simulink model "Kinct_object_tracking"  (Simulink 8.5)
settings: Solver=FixedStepDiscrete  StartTime=0.0  StopTime=inf  RelTol=1e-3
undefined symbols (not defined in the file): HDTV, Rec, strel
libraries: visionsources x3, nid_lib x3, visionsinks x2, simulink x2, visiontextngfix x2, visionstatistics x1, visionconversions x1, visionmorphops x1
settings Model: Creator=Arathos  LastModifiedBy=Arathos_II
settings SolverCC: PositivePriorityOrder=on
settings DataIOCC: SignalLoggingSaveFormat=Dataset
settings OptimizationCC: EnhancedBackFolding=on  SimCompilerOptimization=on
settings DebuggingCC: AlgebraicLoopMsg=none  SolverPrmCheckMsg=warning  FcnCallInpInsideContextMsg=EnableAllAsError
settings RTWCC: RTWCompilerOptimization=on
settings GRTTargetCC: CombineOutputUpdateFcns=on  GRTInterface=off
settings ConfigComp: Description=Design Verifier Custom Configuration Component  DVMaxTestCaseSteps=500  DVTestSuiteOptimization=CombinedObjectives (Nonlinear Extended)  DVDetectActiveLogic=on

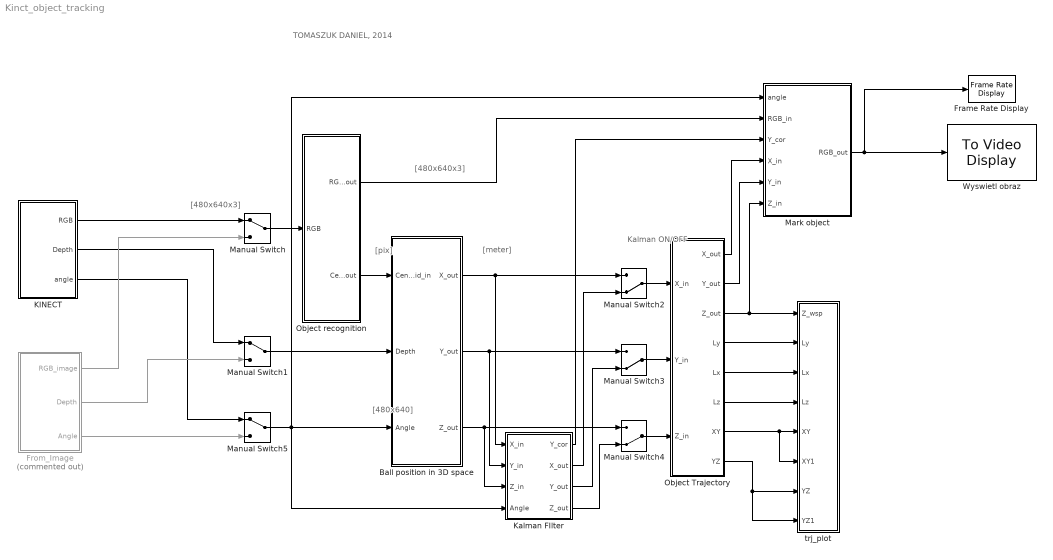
== system Kinct_object_tracking ==
  note: TOMASZUK DANIEL, 2014
  note: Kalman ON/OFF
  note: [meter]
  note: [pix]
  note: [480x640]
  note: [480x640x3]
  note: [480x640x3]
  Ball position in 3D space : Subsystem
  Frame Rate Display : visionsinks/Frame Rate Display  UpdateRate=10
  From_Image : Subsystem  Commented=on
  KINECT : Subsystem
  Kalman FIlter : Subsystem
  Manual Switch : ManualSwitch
  Manual Switch1 : ManualSwitch
  Manual Switch2 : ManualSwitch  CurrentSetting=0
  Manual Switch3 : ManualSwitch  CurrentSetting=0
  Manual Switch4 : ManualSwitch  CurrentSetting=0
  Manual Switch5 : ManualSwitch
  Mark object : Subsystem
  Object Trajectory : Subsystem
  Object recognition : Subsystem
  Wyswietl obraz : visionsinks/To Video Display  windowSizeMode=True size (1:1)  openAtMdlStart=on  fullScreen=off  videoWindowX=411  videoWindowY=172  saveWindowSize=off  videoWindowWidth=640  videoWindowHeight=480  inputColorFormat=RGB  inputType=Obsolete  imagePorts=One multidimensional signal  OutputDevice=On-screen video monitor  dataOrg=Column-major  isWindowOpen=on
  trj_plot : Subsystem
  wires:
  Object Trajectory/3(Z_out) -> trj_plot/1(Z_wsp), Mark object/6(Z_in)
  Object Trajectory/1(X_out) -> Mark object/4(X_in)
  Object Trajectory/2(Y_out) -> Mark object/5(Y_in)
  Object recognition/2(Centroid_out) -> Ball position in 3D space/1(Centroid_in)
  Object recognition/1(RGB_out) -> Mark object/2(RGB_in)
  Manual Switch5/1 -> Ball position in 3D space/3(Angle), Kalman FIlter/4(Angle), Mark object/1(angle)
  From_Image/3(Angle) -> Manual Switch5/2
  KINECT/3(angle) -> Manual Switch5/1
  From_Image/2(Depth) -> Manual Switch1/2
  KINECT/2(Depth) -> Manual Switch1/1
  From_Image/1(RGB_image) -> Manual Switch/2
  KINECT/1(RGB) -> Manual Switch/1
  Mark object/1(RGB_out) -> Wyswietl obraz/1, Frame Rate Display/1
  Manual Switch1/1 -> Ball position in 3D space/2(Depth)
  Manual Switch/1 -> Object recognition/1(RGB)
  Ball position in 3D space/1(X_out) -> Manual Switch2/1, Kalman FIlter/1(X_in)
  Ball position in 3D space/2(Y_out) -> Manual Switch3/1, Kalman FIlter/2(Y_in)
  Ball position in 3D space/3(Z_out) -> Manual Switch4/1, Kalman FIlter/3(Z_in)
  Kalman FIlter/2(X_out) -> Manual Switch2/2
  Kalman FIlter/3(Y_out) -> Manual Switch3/2
  Kalman FIlter/4(Z_out) -> Manual Switch4/2
  Kalman FIlter/1(Y_cor) -> Mark object/3(Y_cor)
  Manual Switch2/1 -> Object Trajectory/1(X_in)
  Manual Switch3/1 -> Object Trajectory/2(Y_in)
  Manual Switch4/1 -> Object Trajectory/3(Z_in)
  Object Trajectory/4(Ly) -> trj_plot/2(Ly)
  Object Trajectory/5(Lx) -> trj_plot/3(Lx)
  Object Trajectory/6(Lz) -> trj_plot/4(Lz)
  Object Trajectory/7(XY) -> trj_plot/6(XY1), trj_plot/5(XY)
  Object Trajectory/8(YZ) -> trj_plot/7(YZ), trj_plot/8(YZ1)

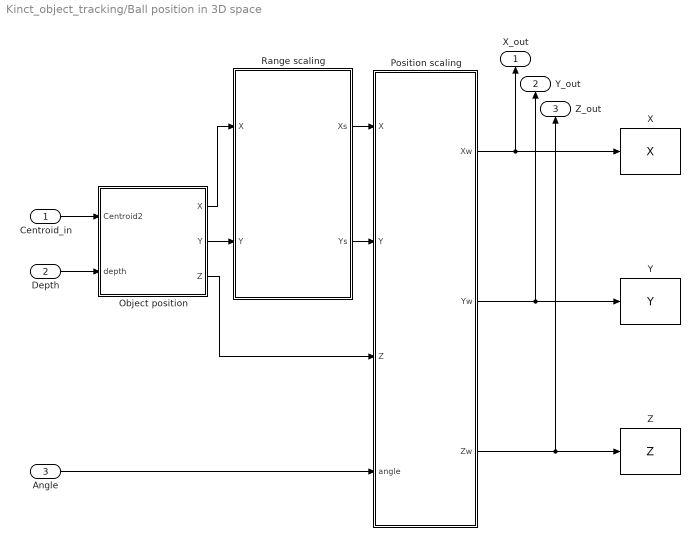
== system Kinct_object_tracking/Ball position in 3D space ==
  Centroid_in : Inport
  Depth : Inport  Port=2
  Angle : Inport  Port=3
  Object position : MATLAB Function  TreatAsAtomicUnit=on
  Position scaling : MATLAB Function  TreatAsAtomicUnit=on
  Range scaling : MATLAB Function  TreatAsAtomicUnit=on
  X : ToWorkspace  VariableName=X  SampleTime=-1
  Y : ToWorkspace  VariableName=Y  SampleTime=-1
  Z : ToWorkspace  VariableName=Z  SampleTime=-1
  X_out : Outport
  Y_out : Outport  Port=2
  Z_out : Outport  Port=3
  wires:
  Object position/3(Z) -> Position scaling/3(Z)
  Object position/1(X) -> Range scaling/1(X)
  Object position/2(Y) -> Range scaling/2(Y)
  Depth/1 -> Object position/2(depth)
  Centroid_in/1 -> Object position/1(Centroid2)
  Position scaling/3(Zw) -> Z_out/1, Z/1
  Range scaling/1(Xs) -> Position scaling/1(X)
  Position scaling/1(Xw) -> X_out/1, X/1
  Range scaling/2(Ys) -> Position scaling/2(Y)
  Position scaling/2(Yw) -> Y_out/1, Y/1
  Angle/1 -> Position scaling/4(angle)

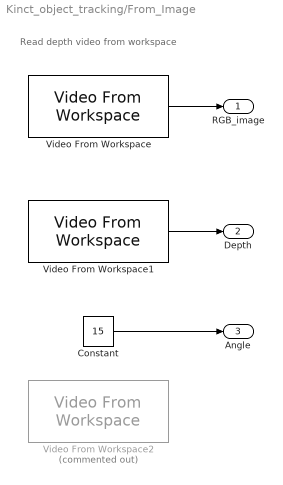
== system Kinct_object_tracking/From_Image ==
  note: Read depth video from workspace
  Constant : Constant  Value=15
  Video From Workspace : visionsources/Video From Workspace  signal=RGB  Ts=0.03333333333333333  finalout=Obsolete  finaloutActive=Holding final value  imagePorts=One multidimensional signal  OutPortLabels=R|G|B
  Video From Workspace1 : visionsources/Video From Workspace  signal=Depth  Ts=0.03333333333333333  finalout=Obsolete  finaloutActive=Holding final value  imagePorts=One multidimensional signal  OutPortLabels=R|G|B
  Video From Workspace2 : visionsources/Video From Workspace  Commented=on  signal=Depth_image  Ts=0.03333333333333333  finalout=Obsolete  finaloutActive=Holding final value  imagePorts=One multidimensional signal  OutPortLabels=R|G|B
  RGB_image : Outport
  Depth : Outport  Port=2
  Angle : Outport  Port=3
  wires:
  Video From Workspace/1 -> RGB_image/1
  Video From Workspace1/1 -> Depth/1
  Constant/1 -> Angle/1

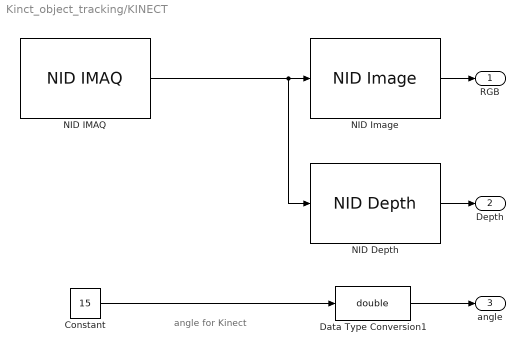
== system Kinct_object_tracking/KINECT ==
  note: angle for Kinect
  Constant : Constant  Value=15
  Data Type Conversion1 : DataTypeConversion  OutDataTypeStr=double  RndMeth=Round
  NID Depth : nid_lib/NID Depth  depthOutput=Depth  conv_XYZ_RW=on  viewer=off
  NID IMAQ : nid_lib/NID IMAQ  imaq_depth=on  imaq_motion=off  imaq_image=on  view_point=on  imaq_skeleton=off  imaq_ir=off  mirror_image=off  imaq_sample_time=1/30  res_fps=QVGA (320x240): 60 FPS  needPsiPose=off  angle_input=off  angle=15  angle_read=off  near_mode=off  seated_mode=off  skeleton_smooth=[0.5 0.5 0.5 0.05 0.04]  infer_skeleton=off
  NID Image : nid_lib/NID Image  imageOutput=RGB
  RGB : Outport
  Depth : Outport  Port=2
  angle : Outport  Port=3
  wires:
  NID IMAQ/1 -> NID Depth/1, NID Image/1
  NID Image/1 -> RGB/1
  Data Type Conversion1/1 -> angle/1
  Constant/1 -> Data Type Conversion1/1
  NID Depth/1 -> Depth/1

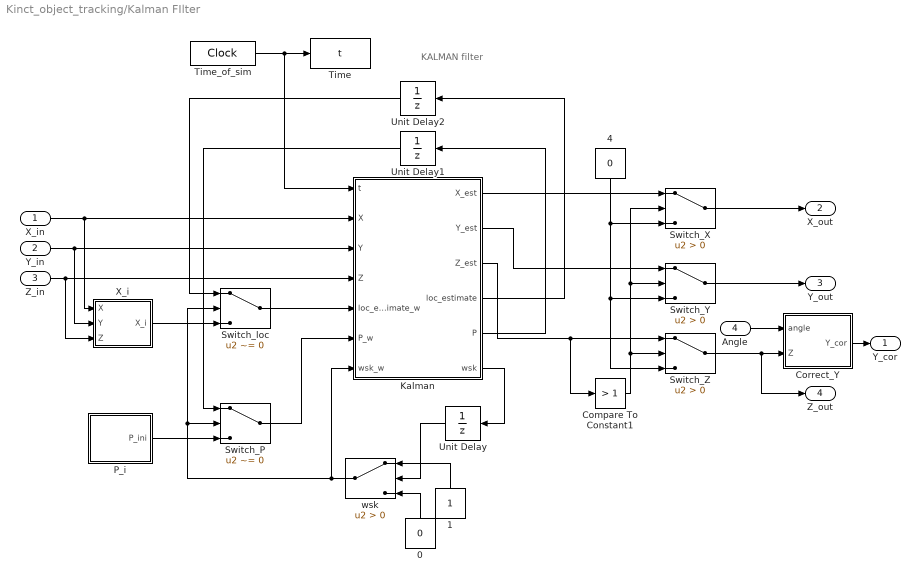
== system Kinct_object_tracking/Kalman FIlter ==
  note: KALMAN filter
  X_in : Inport
  Y_in : Inport  Port=2
  Z_in : Inport  Port=3
  Angle : Inport  Port=4
  0 : Constant  Value=0
  1 : Constant
  4 : Constant  Value=0
  Compare To Constant1 : simulink/Logic and Bit Operations/Compare To Constant  relop=>  const=1  OutDataTypeStr=boolean
  Correct_Y : MATLAB Function  TreatAsAtomicUnit=on
  Kalman : MATLAB Function  TreatAsAtomicUnit=on
  P_i : MATLAB Function  TreatAsAtomicUnit=on
  Switch_P : Switch  Criteria=u2 ~= 0
  Switch_X : Switch  Criteria=u2 > Threshold
  Switch_Y : Switch  Criteria=u2 > Threshold
  Switch_Z : Switch  Criteria=u2 > Threshold
  Switch_loc : Switch  Criteria=u2 ~= 0
  Time : ToWorkspace  VariableName=t  SampleTime=-1
  Time_of_sim : DigitalClock  SampleTime=0.0333333333333333333333333
  Unit Delay : UnitDelay  SampleTime=-1
  Unit Delay1 : UnitDelay  SampleTime=-1
  Unit Delay2 : UnitDelay  SampleTime=-1
  X_i : MATLAB Function  TreatAsAtomicUnit=on
  wsk : Switch  Criteria=u2 > Threshold
  Y_cor : Outport
  X_out : Outport  Port=2
  Y_out : Outport  Port=3
  Z_out : Outport  Port=4
  wires:
  Z_in/1 -> Kalman/4(Z), X_i/3(Z)
  X_in/1 -> X_i/1(X), Kalman/2(X)
  Time_of_sim/1 -> Kalman/1(t), Time/1
  Kalman/4(loc_estimate) -> Unit Delay2/1
  Kalman/5(P) -> Unit Delay1/1
  Kalman/6(wsk) -> Unit Delay/1
  Unit Delay/1 -> wsk/2
  wsk/1 -> Switch_P/2, Switch_loc/2, Kalman/7(wsk_w)
  0/1 -> wsk/3
  1/1 -> wsk/1
  Switch_P/1 -> Kalman/6(P_w)
  P_i/1(P_ini) -> Switch_P/3
  Unit Delay1/1 -> Switch_P/1
  X_i/1(X_i) -> Switch_loc/3
  Switch_loc/1 -> Kalman/5(loc_estimate_w)
  Unit Delay2/1 -> Switch_loc/1
  Y_in/1 -> X_i/2(Y), Kalman/3(Y)
  Switch_X/1 -> X_out/1
  Switch_Y/1 -> Y_out/1
  Correct_Y/1(Y_cor) -> Y_cor/1
  Compare To Constant1/1 -> Switch_X/2, Switch_Y/2, Switch_Z/2
  4/1 -> Switch_Y/3, Switch_Z/3, Switch_X/3
  Angle/1 -> Correct_Y/1(angle)
  Switch_Z/1 -> Z_out/1, Correct_Y/2(Z)
  Kalman/1(X_est) -> Switch_X/1
  Kalman/2(Y_est) -> Switch_Y/1
  Kalman/3(Z_est) -> Compare To Constant1/1, Switch_Z/1

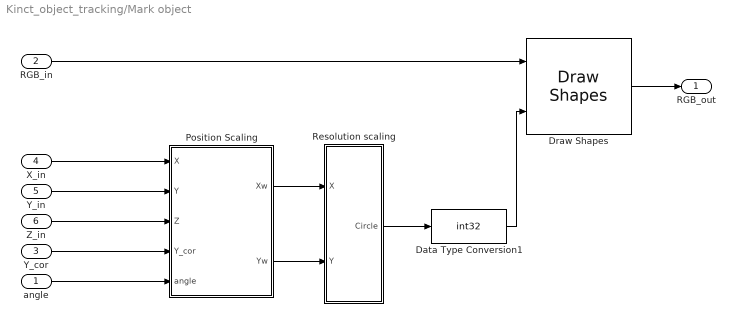
== system Kinct_object_tracking/Mark object ==
  angle : Inport
  RGB_in : Inport  Port=2
  Y_cor : Inport  Port=3
  X_in : Inport  Port=4
  Y_in : Inport  Port=5
  Z_in : Inport  Port=6
  Data Type Conversion1 : DataTypeConversion  OutDataTypeStr=int32  RndMeth=Round
  Draw Shapes : visiontextngfix/Draw Shapes  shape=Circles  fill=off  lineWidth=1  fillClrSource=Specify via dialog  display=User-specified value  intensity=200  color=[0 255 0]  opacity=0.6  viewport=Entire image  antialiasing=off  inType=Obsolete  imagePorts=One multidimensional signal  prodOutputMode=Binary point scaling  prodOutputWordLength=32  prodOutputFracLength=14  memoryMode=Specify word length  memoryWordLength=16  memoryFracLength=14  roundingMode=Floor  overflowMode=off
  Position Scaling : MATLAB Function  TreatAsAtomicUnit=on
  Resolution scaling : MATLAB Function  TreatAsAtomicUnit=on
  RGB_out : Outport
  wires:
  Y_in/1 -> Position Scaling/2(Y)
  X_in/1 -> Position Scaling/1(X)
  RGB_in/1 -> Draw Shapes/1
  Position Scaling/1(Xw) -> Resolution scaling/1(X)
  Position Scaling/2(Yw) -> Resolution scaling/2(Y)
  Resolution scaling/1(Circle) -> Data Type Conversion1/1
  Data Type Conversion1/1 -> Draw Shapes/2
  Draw Shapes/1 -> RGB_out/1
  Z_in/1 -> Position Scaling/3(Z)
  Y_cor/1 -> Position Scaling/4(Y_cor)
  angle/1 -> Position Scaling/5(angle)

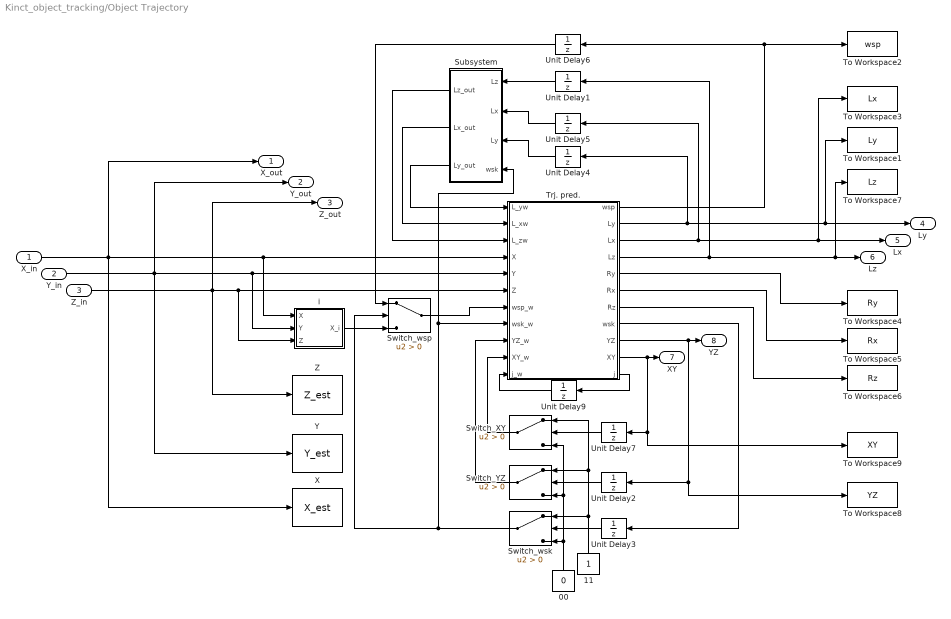
== system Kinct_object_tracking/Object Trajectory ==
  X_in : Inport
  Y_in : Inport  Port=2
  Z_in : Inport  Port=3
  00 : Constant  Value=0
  11 : Constant
  Subsystem : Subsystem
  Switch_XY : Switch  Criteria=u2 > Threshold
  Switch_YZ : Switch  Criteria=u2 > Threshold
  Switch_wsk : Switch  Criteria=u2 > Threshold
  Switch_wsp : Switch  Criteria=u2 > Threshold
  To Workspace1 : ToWorkspace  VariableName=Ly  SampleTime=-1
  To Workspace2 : ToWorkspace  VariableName=wsp  SampleTime=-1
  To Workspace3 : ToWorkspace  VariableName=Lx  SampleTime=-1
  To Workspace4 : ToWorkspace  VariableName=Ry  SampleTime=-1
  To Workspace5 : ToWorkspace  VariableName=Rx  SampleTime=-1
  To Workspace6 : ToWorkspace  VariableName=Rz  SampleTime=-1
  To Workspace7 : ToWorkspace  VariableName=Lz  SampleTime=-1
  To Workspace8 : ToWorkspace  VariableName=YZ  SampleTime=-1
  To Workspace9 : ToWorkspace  VariableName=XY  SampleTime=-1
  Trj. pred. : MATLAB Function  TreatAsAtomicUnit=on
  Unit Delay{1..7,9} (8 alike) : UnitDelay  SampleTime=-1
  X : ToWorkspace  VariableName=X_est  SampleTime=-1
  Y : ToWorkspace  VariableName=Y_est  SampleTime=-1
  Z : ToWorkspace  VariableName=Z_est  SampleTime=-1
  i : MATLAB Function  TreatAsAtomicUnit=on
  X_out : Outport
  Y_out : Outport  Port=2
  Z_out : Outport  Port=3
  Ly : Outport  Port=4
  Lx : Outport  Port=5
  Lz : Outport  Port=6
  XY : Outport  Port=7
  YZ : Outport  Port=8
  wires:
  Trj. pred./2(Ly) -> Unit Delay4/1, To Workspace1/1, Ly/1
  Switch_wsp/1 -> Trj. pred./7(wsp_w)
  Unit Delay6/1 -> Switch_wsp/1
  Trj. pred./11(j) -> Unit Delay9/1
  Unit Delay9/1 -> Trj. pred./11(j_w)
  i/1(X_i) -> Switch_wsp/3
  Trj. pred./3(Lx) -> Unit Delay5/1, Lx/1, To Workspace3/1
  Trj. pred./1(wsp) -> To Workspace2/1, Unit Delay6/1
  Trj. pred./5(Ry) -> To Workspace4/1
  Trj. pred./6(Rx) -> To Workspace5/1
  X_in/1 -> X_out/1, X/1, i/1(X), Trj. pred./4(X)
  Y_in/1 -> Y/1, Y_out/1, i/2(Y), Trj. pred./5(Y)
  Z_in/1 -> Z/1, Z_out/1, i/3(Z), Trj. pred./6(Z)
  Trj. pred./7(Rz) -> To Workspace6/1
  Trj. pred./4(Lz) -> Unit Delay1/1, To Workspace7/1, Lz/1
  Trj. pred./9(YZ) -> Unit Delay2/1, To Workspace8/1, YZ/1
  Trj. pred./8(wsk) -> Unit Delay3/1
  Unit Delay3/1 -> Switch_wsk/2
  Unit Delay2/1 -> Switch_YZ/2
  Unit Delay7/1 -> Switch_XY/2
  Switch_wsk/1 -> Switch_wsp/2, Subsystem/4(wsk), Trj. pred./8(wsk_w)
  Switch_XY/1 -> Trj. pred./10(XY_w)
  Switch_YZ/1 -> Trj. pred./9(YZ_w)
  11/1 -> Switch_wsk/1, Switch_YZ/1, Switch_XY/1
  00/1 -> Switch_wsk/3, Switch_YZ/3, Switch_XY/3
  Trj. pred./10(XY) -> Unit Delay7/1, To Workspace9/1, XY/1
  Unit Delay1/1 -> Subsystem/1(Lz)
  Unit Delay5/1 -> Subsystem/2(Lx)
  Unit Delay4/1 -> Subsystem/3(Ly)
  Subsystem/1(Lz_out) -> Trj. pred./3(L_zw)
  Subsystem/2(Lx_out) -> Trj. pred./2(L_xw)
  Subsystem/3(Ly_out) -> Trj. pred./1(L_yw)

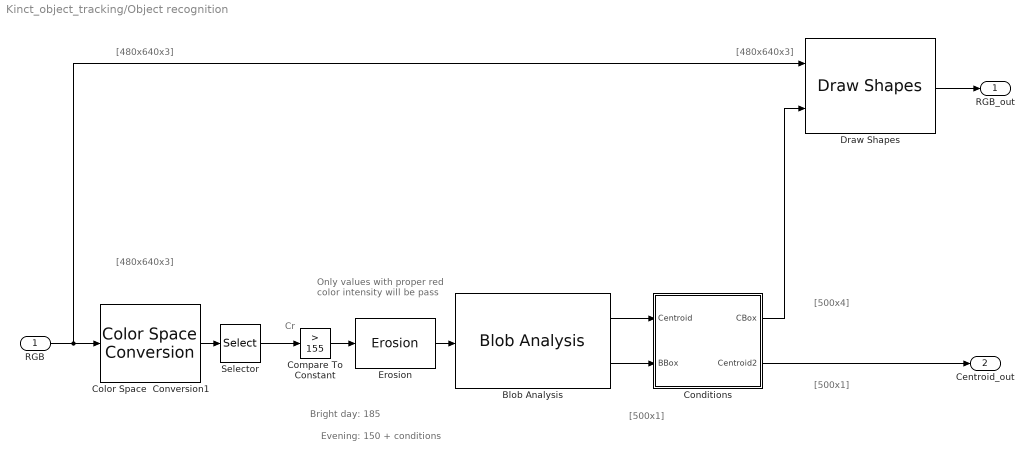
== system Kinct_object_tracking/Object recognition ==
  note: Evening: 150 + conditions
  note: Bright day: 185
  note: [500x4]
  note: Only values with proper red color intensity will be pass
  note: Cr
  note: [500x1]
  note: [500x1]
  note: [480x640x3]
  note: [480x640x3]
  note: [480x640x3]
  RGB : Inport
  Blob Analysis : visionstatistics/Blob Analysis  Tag=vipblks_row_conv  area=off  centroid=on  bBox=on  majorAxis=off  minorAxis=off  angle=off  eccentricity=off  equivDiameterSq=off  extent=off  perimeter=off  maxBlobs=100  warnIfNumBlobsExceeded=on  isCount=off  useMinArea=on  minArea=50  useMaxArea=off  maxArea=3000  excludeBorderBlob=on  outDT=double  isOutVarDim=off  isFill=on  fillValues=-1  conn=8  isLabel=off  outputMode=Binary point scaling  outputWordLength=32  outputFracLength=16  firstCoeffMode=Binary point scaling  firstCoeffWordLength=16  firstCoeffFracLength=14  secondCoeffMode=Binary point scaling  secondCoeffWordLength=32  secondCoeffFracLength=16  accumMode=Binary point scaling  accumWordLength=32  accumFracLength=0  prodOutputMode=Binary point scaling  prodOutputWordLength=32  prodOutputFracLength=16  roundingMode=Floor  overflowMode=off
  Color Space  Conversion1 : visionconversions/Color Space  Conversion  conversion=Obsolete  conversionActive=R'G'B' to Y'CbCr  wp_str=D65  rec=Rec. 709 (HDTV)  sys=1250/50/2:1  imagePorts=One multidimensional signal
  Compare To Constant : simulink/Logic and Bit Operations/Compare To Constant  relop=>  const=155  OutDataTypeStr=boolean
  Conditions : MATLAB Function  TreatAsAtomicUnit=on
  Draw Shapes : visiontextngfix/Draw Shapes  shape=Rectangles  fill=off  lineWidth=1  fillClrSource=Specify via dialog  display=User-specified value  intensity=200  color=[0 0 255]  opacity=0.6  viewport=Entire image  antialiasing=off  inType=Obsolete  imagePorts=One multidimensional signal  prodOutputMode=Binary point scaling  prodOutputWordLength=32  prodOutputFracLength=14  memoryMode=Specify word length  memoryWordLength=16  memoryFracLength=15  roundingMode=Floor  overflowMode=off
  Erosion : visionmorphops/Erosion  nhoodsrc=Specify via dialog  strel=strel('square',4)
  Selector : Selector  NumberOfDimensions=3  InputPortWidth=3  IndexOptions=Select all,Select all,Index vector (dialog)  Indices=[1 3],1,3  OutputSizes=1,1,1
  RGB_out : Outport
  Centroid_out : Outport  Port=2
  wires:
  Erosion/1 -> Blob Analysis/1
  Color Space  Conversion1/1 -> Selector/1
  Blob Analysis/2 -> Conditions/2(BBox)
  Selector/1 -> Compare To Constant/1
  Blob Analysis/1 -> Conditions/1(Centroid)
  RGB/1 -> Draw Shapes/1, Color Space  Conversion1/1
  Compare To Constant/1 -> Erosion/1
  Conditions/2(Centroid2) -> Centroid_out/1
  Conditions/1(CBox) -> Draw Shapes/2
  Draw Shapes/1 -> RGB_out/1

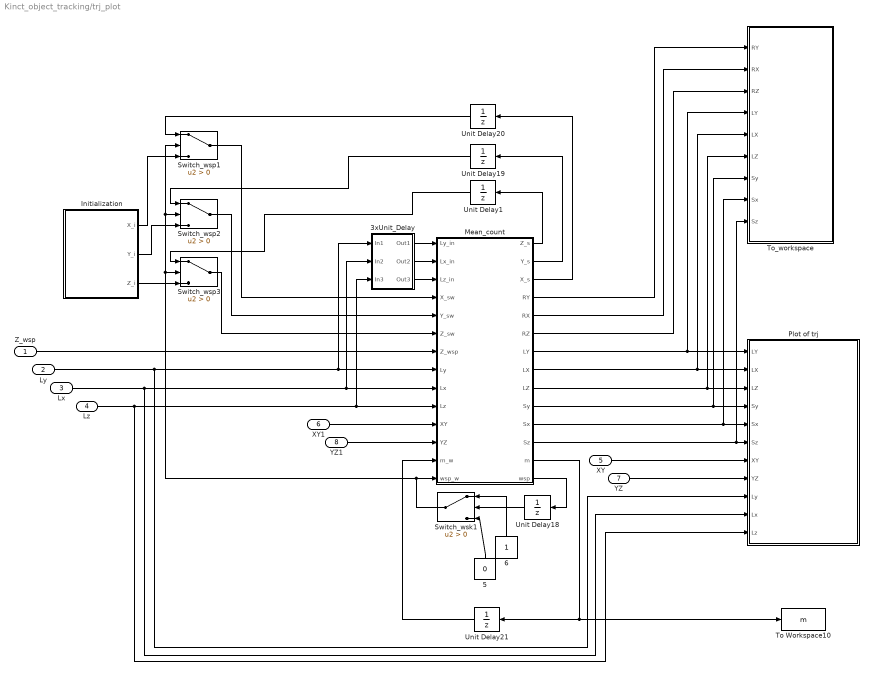
== system Kinct_object_tracking/trj_plot ==
  Z_wsp : Inport
  Ly : Inport  Port=2
  Lx : Inport  Port=3
  Lz : Inport  Port=4
  XY : Inport  Port=5
  XY1 : Inport  Port=6
  YZ : Inport  Port=7
  YZ1 : Inport  Port=8
  3xUnit_Delay : Subsystem
  5 : Constant  Value=0
  6 : Constant
  Initialization : MATLAB Function  TreatAsAtomicUnit=on
  Mean_count : MATLAB Function  TreatAsAtomicUnit=on
  Plot of trj : MATLAB Function  TreatAsAtomicUnit=on
  Switch_wsk1 : Switch  Criteria=u2 > Threshold
  Switch_wsp1 : Switch  Criteria=u2 > Threshold
  Switch_wsp2 : Switch  Criteria=u2 > Threshold
  Switch_wsp3 : Switch  Criteria=u2 > Threshold
  To Workspace10 : ToWorkspace  VariableName=m  SampleTime=-1
  To_workspace : Subsystem
  Unit Delay{1,18..21} (5 alike) : UnitDelay  SampleTime=-1
  wires:
  Lx/1 -> 3xUnit_Delay/2(In2), Mean_count/9(Lx), Plot of trj/10(Lx)
  Ly/1 -> 3xUnit_Delay/1(In1), Mean_count/8(Ly), Plot of trj/9(Ly)
  Mean_count/13(m) -> Unit Delay21/1, To Workspace10/1
  Unit Delay21/1 -> Mean_count/13(m_w)
  Unit Delay18/1 -> Switch_wsk1/2
  5/1 -> Switch_wsk1/3
  6/1 -> Switch_wsk1/1
  Mean_count/14(wsp) -> Unit Delay18/1
  Switch_wsk1/1 -> Mean_count/14(wsp_w), Switch_wsp3/2, Switch_wsp1/2, Switch_wsp2/2
  Mean_count/2(Y_s) -> Unit Delay19/1
  Mean_count/3(X_s) -> Unit Delay20/1
  Unit Delay19/1 -> Switch_wsp2/1
  Unit Delay20/1 -> Switch_wsp1/1
  Initialization/1(X_i) -> Switch_wsp1/3
  Initialization/2(Y_i) -> Switch_wsp2/3
  Switch_wsp1/1 -> Mean_count/4(X_sw)
  Switch_wsp2/1 -> Mean_count/5(Y_sw)
  Mean_count/10(Sy) -> Plot of trj/4(Sy), To_workspace/7(Sy)
  Mean_count/11(Sx) -> To_workspace/8(Sx), Plot of trj/5(Sx)
  Mean_count/7(LY) -> To_workspace/4(LY), Plot of trj/1(LY)
  Mean_count/8(LX) -> To_workspace/5(LX), Plot of trj/2(LX)
  Lz/1 -> 3xUnit_Delay/3(In3), Mean_count/10(Lz), Plot of trj/11(Lz)
  3xUnit_Delay/1(Out1) -> Mean_count/1(Ly_in)
  3xUnit_Delay/2(Out2) -> Mean_count/2(Lx_in)
  3xUnit_Delay/3(Out3) -> Mean_count/3(Lz_in)
  Mean_count/9(LZ) -> To_workspace/6(LZ), Plot of trj/3(LZ)
  Mean_count/12(Sz) -> Plot of trj/6(Sz), To_workspace/9(Sz)
  Initialization/3(Z_i) -> Switch_wsp3/3
  Mean_count/1(Z_s) -> Unit Delay1/1
  Unit Delay1/1 -> Switch_wsp3/1
  Z_wsp/1 -> Mean_count/7(Z_wsp)
  Switch_wsp3/1 -> Mean_count/6(Z_sw)
  XY/1 -> Plot of trj/7(XY)
  YZ/1 -> Plot of trj/8(YZ)
  YZ1/1 -> Mean_count/12(YZ)
  XY1/1 -> Mean_count/11(XY)
  Mean_count/4(RY) -> To_workspace/1(RY)
  Mean_count/5(RX) -> To_workspace/2(RX)
  Mean_count/6(RZ) -> To_workspace/3(RZ)

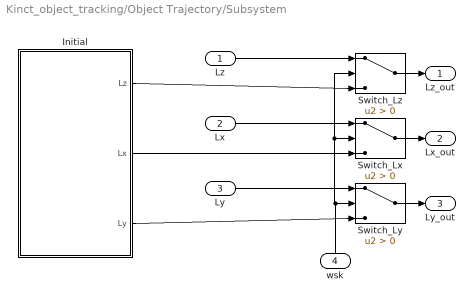
== system Kinct_object_tracking/Object Trajectory/Subsystem ==
  Lz : Inport
  Lx : Inport  Port=2
  Ly : Inport  Port=3
  wsk : Inport  Port=4
  Initial : MATLAB Function  TreatAsAtomicUnit=on
  Switch_Lx : Switch  Criteria=u2 > Threshold
  Switch_Ly : Switch  Criteria=u2 > Threshold
  Switch_Lz : Switch  Criteria=u2 > Threshold
  Lz_out : Outport
  Lx_out : Outport  Port=2
  Ly_out : Outport  Port=3
  wires:
  Switch_Lx/1 -> Lx_out/1
  Ly/1 -> Switch_Ly/1
  Switch_Lz/1 -> Lz_out/1
  Switch_Ly/1 -> Ly_out/1
  wsk/1 -> Switch_Lz/2, Switch_Lx/2, Switch_Ly/2
  Lz/1 -> Switch_Lz/1
  Lx/1 -> Switch_Lx/1
  Initial/1(Lz) -> Switch_Lz/3
  Initial/2(Lx) -> Switch_Lx/3
  Initial/3(Ly) -> Switch_Ly/3

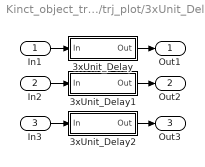
== system Kinct_object_tracking/trj_plot/3xUnit_Delay ==
  In1 : Inport
  In2 : Inport  Port=2
  In3 : Inport  Port=3
  3xUnit_Delay : Subsystem
  3xUnit_Delay1 : Subsystem
  3xUnit_Delay2 : Subsystem
  Out1 : Outport
  Out2 : Outport  Port=2
  Out3 : Outport  Port=3
  wires:
  3xUnit_Delay1/1(Out) -> Out2/1
  In1/1 -> 3xUnit_Delay/1(In)
  In2/1 -> 3xUnit_Delay1/1(In)
  3xUnit_Delay/1(Out) -> Out1/1
  3xUnit_Delay2/1(Out) -> Out3/1
  In3/1 -> 3xUnit_Delay2/1(In)

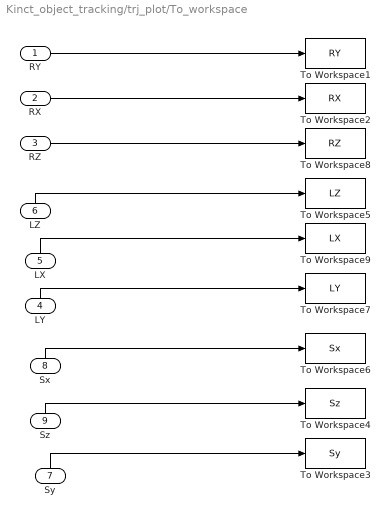
== system Kinct_object_tracking/trj_plot/To_workspace ==
  RY : Inport
  RX : Inport  Port=2
  RZ : Inport  Port=3
  LY : Inport  Port=4
  LX : Inport  Port=5
  LZ : Inport  Port=6
  Sy : Inport  Port=7
  Sx : Inport  Port=8
  Sz : Inport  Port=9
  To Workspace1 : ToWorkspace  VariableName=RY  SampleTime=-1
  To Workspace2 : ToWorkspace  VariableName=RX  SampleTime=-1
  To Workspace3 : ToWorkspace  VariableName=Sy  SampleTime=-1
  To Workspace4 : ToWorkspace  VariableName=Sz  SampleTime=-1
  To Workspace5 : ToWorkspace  VariableName=LZ  SampleTime=-1
  To Workspace6 : ToWorkspace  VariableName=Sx  SampleTime=-1
  To Workspace7 : ToWorkspace  VariableName=LY  SampleTime=-1
  To Workspace8 : ToWorkspace  VariableName=RZ  SampleTime=-1
  To Workspace9 : ToWorkspace  VariableName=LX  SampleTime=-1
  wires:
  Sy/1 -> To Workspace3/1
  LY/1 -> To Workspace7/1
  Sx/1 -> To Workspace6/1
  LZ/1 -> To Workspace5/1
  LX/1 -> To Workspace9/1
  Sz/1 -> To Workspace4/1
  RZ/1 -> To Workspace8/1
  RX/1 -> To Workspace2/1
  RY/1 -> To Workspace1/1

== system Kinct_object_tracking/trj_plot/3xUnit_Delay/3xUnit_Delay ==
  In : Inport
  Unit Delay3 : UnitDelay  SampleTime=-1
  Unit Delay6 : UnitDelay  SampleTime=-1
  Unit Delay7 : UnitDelay  SampleTime=-1
  Out : Outport
  wires:
  In/1 -> Unit Delay7/1
  Unit Delay6/1 -> Out/1
  Unit Delay7/1 -> Unit Delay3/1
  Unit Delay3/1 -> Unit Delay6/1

== system Kinct_object_tracking/trj_plot/3xUnit_Delay/3xUnit_Delay1 ==
  In : Inport
  Unit Delay3 : UnitDelay  SampleTime=-1
  Unit Delay6 : UnitDelay  SampleTime=-1
  Unit Delay7 : UnitDelay  SampleTime=-1
  Out : Outport
  wires:
  In/1 -> Unit Delay7/1
  Unit Delay6/1 -> Out/1
  Unit Delay7/1 -> Unit Delay3/1
  Unit Delay3/1 -> Unit Delay6/1

== system Kinct_object_tracking/trj_plot/3xUnit_Delay/3xUnit_Delay2 ==
  In : Inport
  Unit Delay3 : UnitDelay  SampleTime=-1
  Unit Delay6 : UnitDelay  SampleTime=-1
  Unit Delay7 : UnitDelay  SampleTime=-1
  Out : Outport
  wires:
  In/1 -> Unit Delay7/1
  Unit Delay6/1 -> Out/1
  Unit Delay7/1 -> Unit Delay3/1
  Unit Delay3/1 -> Unit Delay6/1

== matlab function Object Trajectory/Subsystem/Initial ==
  data: Lz output double; Lx output double; Ly output double
function  [Lz,Lx,Ly]= Initial
%#codegen

Lx = [0,0,0];
Ly = [0,0,0];
Lz = [0,0,0];

end

== matlab function Ball position in 3D space/Position scaling ==
  data: Xw output double; X input double; Y input double; Yw output double; Z input double; Zw output double; angle input double
function [Xw, Yw, Zw]  = pos_scaling(X, Y, Z, angle)

% minimal field of viev for X and Y if Z = 0.8m
% Xm = 0.87;
% Ym = 0.63;
Zm = 0.8;
res_m = 0.0013;     % minimal resolution m/pixel

% corection of resolution is counted in dependance of kinect angle
angle_r = (pi/180)*angle;
Y_cor = sin(angle_r)*Z;


% Zm2 = 1.355;
% Rx = 0.660;
% Ry = 0.565;


if (X~=-1 && Y~=-1 && Z~=-1)
    
    % resolution for any Z
    res = (Z/Zm)*res_m;

    % field of view for any Z
    % X_fov = (Z/Zm)*Xm;
    % Y_fov = (Z/Zm)*Ym;
    % 
    % X_rfov = (Z/Zm2).*Rx./res;
    % Y_rfov = (Z/Zm2).*Ry./res;

    Xw = X*res;
    Yw = Y*res;
    Zw = Z;
    

    if angle > 0
     Yw = Yw + Y_cor;
    elseif angle < 0
     Yw = Yw - Y_cor;
    elseif angle == 0
     Yw = Yw;
    end   
else
    Xw = 320;
    Yw = 240;
    Zw = 0;
    % X_rfov = 0;
    % Y_rfov = 0;
end



% looking for objects only for Z>1 and Z<3.5
if Zw > 1 && Zw < 3.5
    Zw = Zw;
    Yw = Yw;
    Xw = Xw;
else
    Xw = 0;
    Yw = 0;
    Zw = 0;
end
end

== matlab function Ball position in 3D space/Range scaling ==
  data: Xs output double; X input double; Y input double; Ys output double
function [Xs, Ys]  = range_scaling(X, Y)


% point (0,0) by default lays in upper left corner of image, 
% transform it to the m iddle of the image
if X ~= 0
    Xs = X - 320;    
else
    Xs = -1;
end

if Y ~= 0
    Ys = -Y + 240;
else
    Ys = -1;
end
end

== matlab function Kalman FIlter/Correct_Y ==
  data: Y_cor output double; angle input double; Z input double
function Y_cor     = corection(angle, Z)
angle_r = (pi/180)*angle;
Y_cor = sin(angle_r)*Z;
end

== matlab function Kalman FIlter/Kalman ==
  data: t input double; X input double; Y input double; Z input double; X_est output double; Y_est output double; Z_est output double; loc_estimate output double; loc_estimate_w input double; P_w input double; P output double; wsk_w input double; wsk output double
function [X_est, Y_est, Z_est,loc_estimate, P, wsk]   = kalman(t,X,Y,Z, loc_estimate_w, P_w, wsk_w)
%% main varaiables
wsk = wsk_w;
t = 30*t + 1;    % matrix index can not be equal to 0 and must be integer 
t = round(t);

dt = 0.1;
u  = 0.05; % 

noise_mag = 2; % process noise for kalman filter


tkn_x = 0.1;  % noise in X
tkn_y = 0.1;  % noise in Y
tkn_z = 0.1;  % noise in Z

% measurement noise
Ez = [tkn_x, 0, 0; 0 tkn_y, 0; 0, 0, tkn_z];

 Ex = [dt^4/4, 0, 0, dt^3/2, 0, 0, 0.5*dt^2, 0, 0; ... 
     0, dt^4/4, 0, 0, dt^3/2, 0,  0, 0.5*dt^2, 0; ...
     0, 0, dt^4/4, 0, 0, dt^3/2, 0,  0,  0.5*dt^2; ...
     dt^3/2, 0, 0, dt^2, 0, 0, dt, 0, 0; ...
     0, dt^3/2, 0, 0, dt^2, 0, 0,  dt, 0; ...
     0, 0, dt^3/2, 0, 0, dt^2, 0, 0, dt; ...
     0.5*dt^2, 0, 0, dt, 0, 0, 1, 0, 0; ...
     0, 0.5*dt^2, 0, 0, dt, 0 , 0 , 1, 0; ...
     0, 0, 0.5*dt^2, 0, 0, dt, 0, 0 , 1].*noise_mag;
%  Ex = ones(9).*noise_mag; 
 
%% (Coefficent matrices): 2nd order equations, description of ball movement
 % state matrix
 A = [1,0, 0, dt, 0, 0, 0.5*dt^2, 0, 0;  ...
     0, 1, 0, 0, dt, 0, 0,  0.5*dt^2, 0;  ...
     0, 0, 1, 0, 0, dt, 0, 0,  0.5*dt^2;  ...
     0, 0, 0, 1, 0, 0, dt, 0, 0;   ...
     0, 0, 0, 0, 1, 0, 0, dt, 0;  ...
     0, 0, 0, 0, 0, 1, 0, 0, dt; ...
     0, 0, 0, 0, 0, 0, 1, 0, 0;   ...
     0, 0, 0, 0, 0, 0, 0, 1, 0;  ...
     0, 0, 0, 0, 0, 0, 0, 0, 1;];  
 

B = [0.5*(dt^2); 0.5*(dt^2); 0.5*(dt^2); dt; dt; dt; 1; 1; 1];

% outputs from kalman filter - positions only
C = [1 0 0 0 0 0 0 0 0; ...
     0 1 0 0 0 0 0 0 0;  ...
     0 0 1 0 0 0 0 0 0]; 

loc_meas = zeros(3,20000);

%% real time loop START____________________________________________________________________________________________________
    P = P_w; % covariance matrix
    
    loc_estimate = loc_estimate_w; % estimated object position
   
    loc_meas(1,t) = X;
    loc_meas(2,t) = Y;
    loc_meas(3,t) = Z;
    
    if loc_estimate(3) ~= 0       % set wsk=1 if object has been recognized
        wsk = 1;
    end

    % if there was index overflow (hasn't been tested)
    if t == 999
            loc_meas = zeros(3,t*100);  
    end    

    %% DO THE KALMAN !! (FILTER)  
    
    % loctaion estimation
    loc_estimate = A * loc_estimate + B*u;

    % next covariance matrix
    P = A * P * A' + Ex;
    
    %  Kalman gain
    K = P*C'*inv(C*P*C'+Ez);
    
    % actualization of object position
    if isnan(loc_meas(1,t)) ~= 1 || isnan(loc_meas(3,t)) ~= 0
        loc_estimate = loc_estimate + K * (loc_meas(:,t) - C * loc_estimate);
    end
    % actualization of covariance matrix
    P =  (eye(9)-K*C)*P;
    % outputs from Kalman
    X_est = loc_estimate(1);
    Y_est = loc_estimate(2);
    Z_est = loc_estimate(3);
    
    
 %% end of loop ________________________________________________________________________________________________


end

== matlab function Kalman FIlter/X_i ==
  data: X_i output double; X input double; Y input double; Z input double
function X_i  = initial(X,Y,Z)

%initial matrix for t=0
X_i = [X; Y; Z; 0; 0; 0; 0; 0; 0];
end

== matlab function Kalman FIlter/P_i ==
  data: P_ini output double
function P_ini  = initial
%#codegen



dt = 0.1;       %(0.1 => 3fps;  0.2 => 6 fps)
noise_mag = 2;  %process noise
 
  Ex = [0.25*dt^4, 0, 0, 0.5*dt^3, 0, 0, 0.5*dt^2, 0, 0; ... 
        0, 0.25*dt^4, 0, 0, 0.5*dt^3, 0, 0,  0.5*dt^2, 0; ...
        0, 0, 0.25*dt^4, 0, 0, 0.5*dt^3, 0,  0,  0.5*dt^2; ...
        0.5*dt^3, 0, 0, dt^2, 0, 0, dt, 0, 0; ...
        0, 0.5*dt^3, 0, 0, dt^2, 0, 0,  dt, 0; ...
        0, 0, 0.5*dt^3, 0, 0, dt^2, 0, 0, dt; ...
        0.5*dt^2, 0, 0, dt, 0, 0, 1, 0, 0; ...
        0, 0.5*dt^2, 0, 0, dt, 0 , 0 , 1, 0; ...
        0, 0, 0.5*dt^2, 0, 0, dt, 0, 0 , 1].*noise_mag;
    
  
 
P_ini = Ex; % covariance matrix

end

== matlab function Object Trajectory/Trj. pred. ==
  data: wsp output double; L_yw input double; L_xw input double; L_zw input double; Ly output double; Lx output double; Lz output double; Ry output double; Rx output double; Rz output double; wsk output double; YZ output double; XY output double; X input double; Y input double; Z input double; wsp_w input double; wsk_w input double; YZ_w input double; XY_w input double; j_w input double; j output double
function [wsp,Ly,Lx,Lz,Ry,Rx,Rz,wsk,YZ,XY,j]   = trj_prediction(L_yw,L_xw,L_zw,X,Y,Z,wsp_w,wsk_w,YZ_w,XY_w,j_w)
%#codegen
Rx = 0;
Ry = 0;
Rz = 0;

YZ = YZ_w;
XY = XY_w;

wsp = wsp_w;
j = j_w;
wsk = wsk_w;

% if object exists
      if  (Z ~=0 && X ~=0 && Y ~=0)
          wsk = 1;
      end

      if wsk ==1 && (Z ~=0 && X ~=0 && Y ~=0)
              
          j = j + 1;
       
          wsp(j,1) = X;
          wsp(j,2) = Y;
          wsp(j,3) = Z; 
          
          % movement in XY or YX axis, Z~const.     
          % X changes in linear manner
          if (abs(wsp(1,1) - wsp(j,1)) >= 0.4) && (abs(wsp(1,2) - wsp(j,2)) >= 0.4)
              XY = 1;
              % polyfit(X,Y,2)          
              [Ly,Rly] = polyfit(wsp(:,1), wsp(:,2),2); 

              % Ry = diag(inv(Rly.R)*inv(Rly.R')).*Rly.normr.^2./Rly.df;
              Ry = 1 - Rly.normr^2 / norm(wsp(:,2)-mean(wsp(:,2)))^2;

              % polyfit(X,Z,2)
              [Lz,Rlz] = polyfit(wsp(:,1), wsp(:,3),2);          

              % Rx = diag(inv(Rlx.R)*inv(Rlx.R')).*Rlx.normr.^2./Rlx.df;
              Rz = 1 - Rlz.normr^2 / norm(wsp(:,3)-mean(wsp(:,3)))^2; 
          else
              Ly = L_yw;              
              Lz = L_zw;
          end
          % movement in YZ or ZY axis, X~const.     
          % Z changes in linear manner
          if (abs(wsp(1,2) - wsp(j,2)) >= 0.4) && (abs(wsp(1,3) - wsp(j,3)) >= 1) && XY ==0  
              YZ = 1;
              % polyfit(Z,Y,2)          
              [Ly,Rly] = polyfit(wsp(:,3), wsp(:,2),2); 

              % Ry = diag(inv(Rly.R)*inv(Rly.R')).*Rly.normr.^2./Rly.df;
              Ry = 1 - Rly.normr^2 / norm(wsp(:,2)-mean(wsp(:,2)))^2;

              % polyfit(Z,X,2)
              [Lx,Rlx] = polyfit(wsp(:,3), wsp(:,1),2);          

              % Rx = diag(inv(Rlx.R)*inv(Rlx.R')).*Rlx.normr.^2./Rlx.df;
              Rx = 1 - Rlx.normr^2 / norm(wsp(:,1)-mean(wsp(:,1)))^2;   
          else              
              Lx = L_xw;
          end
          
          
          % if movement in every axis
          if (abs(wsp(1,2) - wsp(j,2)) >= 0.4) && (abs(wsp(1,3) - wsp(j,3)) >= 1) && ...
             (abs(wsp(1,1) - wsp(j,1)) >= 0.4) 
              YZ = 1;
              XY = 1;
              % polyfit(Z,Y,2)          
              [Ly,Rly] = polyfit(wsp(:,3), wsp(:,2),2); 

              % Ry = diag(inv(Rly.R)*inv(Rly.R')).*Rly.normr.^2./Rly.df;
              Ry = 1 - Rly.normr^2 / norm(wsp(:,2)-mean(wsp(:,2)))^2;

              % polyfit(Z,X,2)
              [Lx,Rlx] = polyfit(wsp(:,3), wsp(:,1),2);          

              % Rx = diag(inv(Rlx.R)*inv(Rlx.R')).*Rlx.normr.^2./Rlx.df;
              Rx = 1 - Rlx.normr^2 / norm(wsp(:,1)-mean(wsp(:,1)))^2;
          end
                
      else
          % if there is no object or object moved from camera
         
          Ly = L_yw;
          Lx = L_xw;
          Lz = L_zw;
          
          j = j_w;
          
          Rz = 0;
          Ry = 0;
          Rx = 0;
      end
end

== matlab function Object Trajectory/i ==
  data: X_i output double; X input double; Y input double; Z input double
function X_i  = initial(X,Y,Z)


X_i = zeros(5000,3);

X_i(:,1) = X;
X_i(:,2) = Y;
X_i(:,3) = Z;

end

== matlab function Mark object/Position Scaling ==
  data: Xw output double; X input double; Y input double; Yw output double; Z input double; Y_cor input double; angle input double
function [Xw, Yw]  = pos_scaling(X, Y, Z, Y_cor, angle)
%#codegen


if X~=-1 && Y~=-1
Xm = 0.87;
Ym = 0.63;
Zm = 0.8;

res_m = 0.0013;     

% X_fov = (Z/Zm)*Xm;
% Y_fov = (Z/Zm)*Ym;

if angle > 0
    Y = Y - Y_cor;
elseif angle < 0 
    Y = Y + Y_cor;
elseif angle == 0
    Y = Y;
end


res = (Z/Zm)*res_m;
Xw = X./res;
Yw = Y./res;


else
Xw = 0;
Yw = 0;
end
end

== matlab function Mark object/Resolution scaling ==
  data: X input double; Y input double; Circle output double
function Circle = scale_1(X, Y)
%#codegen

    Xs = X + 320;
    Ys = -Y + 240;

Circle = [ Xs; Ys; 10];


end

== matlab function trj_plot/Mean_count ==
  data: Z_s output double; Ly_in input double; Lx_in input double; Lz_in input double; Y_s output double; X_sw input double; Y_sw input double; X_s output double; RY output double; RX output double; RZ output double; LY output double; LX output double; LZ output double; Sy output double; Sx output double; Sz output double; Z_sw input double; Z_wsp input double; Ly input double; Lx input double; Lz input double; XY input double; YZ input double; m output double; m_w input double; wsp output double; wsp_w input double
function [Z_s, Y_s, X_s, RY, RX, RZ, LY, LX, LZ, Sy, Sx, Sz, m, wsp] = mean_count(Ly_in, Lx_in, Lz_in, X_sw, Y_sw,Z_sw, Z_wsp, Ly, Lx, Lz,XY,YZ,m_w,wsp_w)
%#codegen

% what kind of movement
if XY == 1 && YZ == 0    
   t1   = -1;
   t2_1 =  1;
else
   t1   = 0;
   t2_1 = 3.5;
end 

RY = 0;
RX = 0;
RZ = 0;
% checking if final trajectory has been obtained and the movement has ended
Sx = (Lx(1,1) - Lx_in(1,1)) + (Lx(1,2) - Lx_in(1,2)) + (Lx(1,3) - Lx_in(1,3));
Sy = (Ly(1,1) - Ly_in(1,1)) + (Ly(1,2) - Ly_in(1,2)) + (Ly(1,3) - Ly_in(1,3));
Sz = (Lz(1,1) - Lz_in(1,1)) + (Lz(1,2) - Lz_in(1,2)) + (Lz(1,3) - Lz_in(1,3));


t = t1:0.1:t2_1;
ts = length(t);

wsp = wsp_w;


Y_s = Y_sw;
X_s = X_sw;
Z_s = Z_sw;

m = m_w;


tt = zeros(ts,1);

Y = zeros(ts,1);
X = zeros(ts,1);
Z = zeros(ts,1);

if (Ly(1,1) < 0 && Z_wsp ~=0) 
    m = m+1;
 
    wsp = 1;
       
    if XY == 1 && YZ == 0    
       t1   = -1;
       t2_1 =  1;
    else
       t1   = 0;
       t2_1 = 3.5;
    end 
      
for t = t1:0.1:t2_1;
 
    if t1 == 0
        t2 = round(10*t)+1;
    else
        t2 = round(10*t)+11;
    end     
    
        Yy = Ly(1,1)*t^2 + Ly(1,2)*t + Ly(1,3);
        Yx = Lx(1,1)*t^2 + Lx(1,2)*t + Lx(1,3);
        Zz = Lz(1,1)*t^2 + Lz(1,2)*t + Lz(1,3); 
        

%     Yy = Ly_tab_in(m,1)*t^2 + Ly_tab_in(m,2)*t + Ly_tab_in(m,3);
%     Yx = Lx_tab_in(m,1)*t^2 + Lx_tab_in(m,2)*t + Lx_tab_in(m,3);
    

    Y_s(t2,m) = Yy; 
    X_s(t2,m) = Yx;
    Z_s(t2,m) = Zz;
   
    % checking for errors
    if ((Ly(1,1) > 0 || Yx > 1 || Yx < -1) && XY == 1) || ((Ly(1,1) > 0 || Yy > 3 || Yy < -3) && YZ == 1)  
        % 
        % 
       if m == 1
            Y_s(t2,m) = Y_s(t2,1); 
            X_s(t2,m) = X_s(t2,1);
            Z_s(t2,m) = Z_s(t2,1);
       else
        % 
            Y_s(t2,m) = Y_s(t2,m-1); 
            X_s(t2,m) = X_s(t2,m-1); 
            Z_s(t2,m) = Z_s(t2,m-1);
       end
        % removing wrong trajectory
            m = m - 1;
        % 
       break      
    else

%             hold on
%             grid on
%             plot(t,Y_s(t2,m),'r-');  
%             plot(t,X_s(t2,m),'b-');
%             plot3(t,X_s(t2,1),Y_s(t2,1), 'g+');
    end            
end
end  




% how many initial trajectory should be omitted when counting final
% trajectory
% 

min = 0;

if m > min && Sx == 0 && Sy == 0 && Sz == 0   
for t = t1:0.1:t2_1; 
    
for k = 1:1:ts    
    if XY == 1 && YZ ==0    
         tt(k,1) = 0.1*k - 1.1;
    else
         tt(k,1) = 0.1*k - 0.1;
    end     
end    
      
    
    if t1 == 0
        ts2 = round(10*t)+1;
    else
        ts2 = round(10*t)+11;
    end    
    % sum
    for i = (min+1):1:m               
       Y(ts2,1) = Y(ts2,1) + Y_s(ts2,i);
       X(ts2,1) = X(ts2,1) + X_s(ts2,i);
       Z(ts2,1) = Z(ts2,1) + Z_s(ts2,i);
    end 
    % div
        Y(ts2,1) = Y(ts2,1)/(m-min);
        X(ts2,1) = X(ts2,1)/(m-min);
        Z(ts2,1) = Z(ts2,1)/(m-min);
end

% coeficients of final trajectory
    [LY,RLY] =  polyfit(tt,Y,2);
    [LX,RLX] =  polyfit(tt,X,2);
    [LZ,RLZ] =  polyfit(tt,Z,2);
    RY = 1 - (RLY.normr^2 / norm(Y(:,1)-mean(Y(:,1)))^2);
    RX = 1 - (RLX.normr^2 / norm(X(:,1)-mean(X(:,1)))^2);
    RZ = 1 - (RLZ.normr^2 / norm(Z(:,1)-mean(Z(:,1)))^2);
else
    LY = [0,0,0];
    LX = [0,0,0];
    LZ = [0,0,0];
end

end

== matlab function trj_plot/Initialization ==
  data: X_i output double; Y_i output double; Z_i output double
function [X_i, Y_i, Z_i]  = initial
    %#codegen
   
    % t = 0:0.1:3.5;
    t = -1:0.1:4;
    ts = length(t);
    Y_i = zeros(ts,100);
    X_i = zeros(ts,100);
    Z_i = zeros(ts,100);
end

== matlab function trj_plot/Plot of trj ==
  data: LY input double; LX input double; LZ input double; Sy input double; Sx input double; Sz input double; XY input double; YZ input double; Ly input double; Lx input double; Lz input double
function     rys(LY, LX, LZ, Sy, Sx, Sz, XY, YZ, Ly, Lx, Lz)
%#codegen

grid on

t = -1:0.1:4;

% object has been detected and already moved
if Sy == 0 && Sx == 0 && Sz == 0
    % 
    Y = LY(1,1).*t.^2 + LY(1,2).*t + LY(1,3);
    X = LX(1,1).*t.^2 + LX(1,2).*t + LX(1,3);
    Z = LZ(1,1).*t.^2 + LZ(1,2).*t + LZ(1,3);
    
    %  
    Y2 = Ly(1,1).*t.^2 + Ly(1,2).*t + Ly(1,3);
    X2 = Lx(1,1).*t.^2 + Lx(1,2).*t + Lx(1,3);
    Z2 = Lz(1,1).*t.^2 + Lz(1,2).*t + Lz(1,3);

   

if XY == 1 && YZ == 0
%% fig. 2D    
%     hold on
%     title('2D')
%     xlabel('X[m]')%     
%     axis([-1 1 -1 3.5])
%     ylabel('Y[m] /  Z[m]')
%     plot(t,Y2,'r-'); 
%     plot(t,Z2,'c-');
%     if LY(1,1) <= 0 
%         plot(t,Z,'b-'); 
%         plot(t,Y,'g-');
%     end

% fig. 3D
    hold on
    axis([-1 1 0 3.5 -1 2 ])
    title(' 3D')
    xlabel(' X[m]')
    ylabel(' Z[m]')
    zlabel(' Y[m]')
    
    if LY(1,1) <= 0
        plot3(t,Z,Y,'g');
    end
    plot3(t,Z2,Y2,'b');

hold off
end    
    
if XY == 0 && YZ == 1
%% rys. 2D    
%     hold on
%     title(' 2D')
%     xlabel(' Z[m]')%     
%     axis([0 3.5 -1 2])
%     ylabel(' Y[m] /  X[m]')
%     plot(t,Y2,'r-'); 
%     plot(t,X2,'c-');
% if LY(1,1) <= 0 
%     plot(t,X,'b-'); 
%     plot(t,Y,'g-');
% end
%  rys. 3D
    hold on
    axis([0 3.5 -1 1 -1 2 ])
    title(' 3D')
    xlabel('Z[m]')
    ylabel('X[m]')
    zlabel('Y[m]')
    
    if LY(1,1) <= 0
        plot3(t,X,Y,'g');
    end
    plot3(t,X2,Y2,'b');
hold off
end
    
if XY == 1 && YZ == 1
%% rys. 2D    
%     hold on
%     title(' 2D')
%     xlabel('Z[m]')     
%     axis([0 3.5 -1 2])
%     ylabel('Y[m] / X[m]')
%     plot(t,Y2,'r-'); 
%     plot(t,X2,'c-');
% if LY(1,1) <= 0
%     plot(t,X,'b-'); 
%     plot(t,Y,'g-');
% end


%% rys. 3D
    hold on
    axis([0 3.5 -1 1 -1 2 ])
    title('3D')
    xlabel('Z[m]')
    ylabel('X[m]')
    zlabel('Y[m]')
    
    if LY(1,1) <= 0
        plot3(t,X,Y,'g');
    end
    plot3(t,X2,Y2,'b');
hold off
end
end
end

== matlab function Object recognition/Conditions ==
  data: Centroid input double; BBox input double; CBox output double; Centroid2 output double
function [CBox, Centroid2] = fcn(Centroid, BBox)
%#codegen

% m = length(a);          % m jest d?ugo?ci wektora osi g?ównej elipsy


CBox = BBox;            % obwiednia elispy
Centroid2 = Centroid;  
  
% Th = 1;
% Th_max = 5000;
% for n = 1:m   
%     
%     % nie s? brane pod uwag? elementy o polu mniejszym
% %     if Area(n) < Th || Area(n) > Th_max
% %         CBox(n,:)=-1;
% %     end
%     
%     
%     % wspó?rz?dne ?rodka elementu (wsp. pikselowe w obrazie)
% %     X = round(Centroid(n,1));
% %     Y = round(Centroid(n,2));
%         
% %     if X > 0 || Y > 0
% %         if Depth(Y,X)==0 || Depth(Y,X) > 10
% %             CBox(n,:)=-1;
% %         end
% %     end
% end


% je?eli który? z warunków nie zosta? spe?niony lub nic nie wykryto
% for n = 1:m
%     if CBox(n,1)==-1
%         Centroid2(n,:)=-1;   
%     end
% end


end

== matlab function Ball position in 3D space/Object position ==
  data: X output double; Y output double; Z output double; Centroid2 input double; depth input double
function [X, Y, Z] = Object_pos(Centroid2, depth)
%#codegen

m = size(Centroid2,1);

X = 0;
Y = 0;
Z = 0;

% Zm = 0.8;
% res_m = 0.0013;     minimal resolution m/pix for Zm
%                      
% roz = 0.025;

for n = 1:m
    if Centroid2(n,1)~=-1;
        % marker position
        % resolution for any Z (m/pix) 
      
%         res = (Z/Zm)*res_m;        
%         if res ==0
%             res = 1;
%         end        
%         Xr = roz/res;
%         Yr = roz/res;  
%         
    % position form RGB image       
    X = round(Centroid2(n,1));  
    Y = round(Centroid2(n,2));
    
    
 % scaling function (if there is no active compensation) 
    if (X > 0 && X < 320) && (Y > 0 && Y < 240)
    % left up:
        X_c = round(1.162711*X - 29.06779);
        Y_c = round(1.101449*Y - 36.3478);

    elseif (X > 320 && X < 640) && (Y > 0 && Y < 240)
    % right up:
        X_c = round(1.12075*X - 16.64);
        Y_c = round(1.101449*Y - 36.3478);

    elseif (X > 0 && X < 320) && (Y > 240 && Y < 480)
    % left down:
        X_c = round(1.162711*X - 29.06779); 
        Y_c = round(1.145454*Y - 46.909090);

    elseif (X > 320 && X < 640) && (Y > 240 && Y < 480)
    % right down:
        X_c = round(1.12075*X - 16.64);
        Y_c = round(1.145454*Y - 46.909090);

    elseif X == 320 && Y == 240
    % middle
        X_c = X + 23;
        Y_c = Y - 12;
    else
        X_c = 0;
        Y_c = 0;
    end
     
    
    if Y_c <= 0 || X_c <= 0
        Y_c = 1;
        X_c = 1;
    end
    
    if Y_c >= 480 || X_c >= 640
        Y_c = 480;
        X_c = 640;
    end
    
% if there is no resolution compensation in NID IMAQ, then use:
% Z = depth(Y_c,X_c); 

  Z = depth(Y,X); 
%         Xz = round(X + Xr);
%         Yz = round(Y - Yr); 
              
    end    
end

% t = size(Tab,3);
% Z = Tab(1,3,t);


end
